simulink model "fk_omni"  (R2015a)
settings: Solver=ode45  StartTime=0.0  StopTime=10.0  RelTol=1e-3
libraries: aerolibutil x5, simulink x1
settings Model: Creator=Pinnacle  LastModifiedBy=Pinnacle

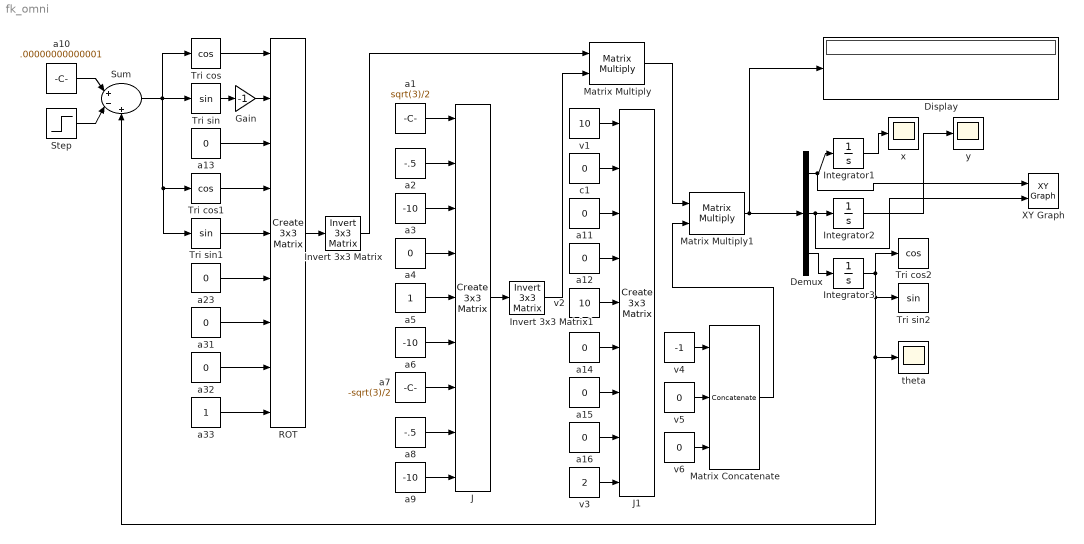
== system fk_omni ==
  Demux : Demux  Outputs=3
  Display : Display
  Gain : Gain  Gain=-1
  Integrator1 : Integrator
  Integrator2 : Integrator
  Integrator3 : Integrator
  Invert 3x3 Matrix : aerolibutil/Invert  3x3 Matrix
  Invert 3x3 Matrix1 : aerolibutil/Invert  3x3 Matrix
  J : aerolibutil/Create 3x3 Matrix
  J1 : aerolibutil/Create 3x3 Matrix
  Matrix Concatenate : Concatenate  NumInputs=3  Mode=Multidimensional array
  Matrix Multiply : Product  Multiplication=Matrix(*)
  Matrix Multiply1 : Product  Multiplication=Matrix(*)
  ROT : aerolibutil/Create 3x3 Matrix
  Step : Step  Time=.00001  After=0.00000000000001  SampleTime=0
  Sum : Sum  Inputs=|+-+
  Tri cos : Trigonometry  Operator=cos
  Tri cos1 : Trigonometry  Operator=cos
  Tri cos2 : Trigonometry  Operator=cos
  Tri sin : Trigonometry
  Tri sin1 : Trigonometry
  Tri sin2 : Trigonometry
  XY Graph : simulink/Sinks/XY Graph  xmin=-100  xmax=100  ymin=-100  ymax=100  st=-1
  a1 : Constant  Value=sqrt(3)/2
  a10 : Constant  Value=.00000000000001
  a{4,11..16,23,31..32} (10 alike) : Constant  Value=0
  a2 : Constant  Value=-.5
  a3 : Constant  Value=-10
  a33 : Constant
  a5 : Constant
  a6 : Constant  Value=-10
  a7 : Constant  Value=-sqrt(3)/2
  a8 : Constant  Value=-.5
  a9 : Constant  Value=-10
  c1 : Constant  Value=0
  theta : Scope
      settings: SaveName=ScopeData2
  v1 : Constant  Value=10
  v2 : Constant  Value=10
  v3 : Constant  Value=2
  v4 : Constant  Value=-1
  v5 : Constant  Value=0
  v6 : Constant  Value=0
  x : Scope
  y : Scope
  wires:
  ROT/1 -> Invert 3x3 Matrix/1
  J/1 -> Invert 3x3 Matrix1/1
  Tri cos/1 -> ROT/1
  a13/1 -> ROT/3
  Tri cos1/1 -> ROT/4
  Tri sin1/1 -> ROT/5
  a23/1 -> ROT/6
  a31/1 -> ROT/7
  a32/1 -> ROT/8
  a33/1 -> ROT/9
  a2/1 -> J/2
  a4/1 -> J/4
  a1/1 -> J/1
  a3/1 -> J/3
  a5/1 -> J/5
  a6/1 -> J/6
  a7/1 -> J/7
  a8/1 -> J/8
  a9/1 -> J/9
  Invert 3x3 Matrix/1 -> Matrix Multiply/1
  v1/1 -> J1/1
  Integrator1/1 -> x/1
  Integrator2/1 -> y/1
  Tri sin/1 -> Gain/1
  Gain/1 -> ROT/2
  a10/1 -> Sum/1
  Sum/1 -> Tri sin1/1, Tri cos1/1, Tri cos/1, Tri sin/1
  Integrator3/1 -> Tri cos2/1, Sum/3, theta/1, Tri sin2/1
  v3/1 -> J1/9
  v2/1 -> J1/5
  c1/1 -> J1/2
  a11/1 -> J1/3
  a12/1 -> J1/4
  a14/1 -> J1/6
  a15/1 -> J1/7
  a16/1 -> J1/8
  Invert 3x3 Matrix1/1 -> Matrix Multiply/2
  Matrix Multiply/1 -> Matrix Multiply1/1
  v4/1 -> Matrix Concatenate/1
  v5/1 -> Matrix Concatenate/2
  v6/1 -> Matrix Concatenate/3
  Matrix Concatenate/1 -> Matrix Multiply1/2
  Matrix Multiply1/1 -> Demux/1, Display/1
  Demux/3 -> Integrator3/1
  Step/1 -> Sum/2
  Demux/1 -> XY Graph/1, Integrator1/1
  Demux/2 -> XY Graph/2, Integrator2/1
